simulink model "Swarm_Robot_Base_2017b"  (R2017b)
settings: Solver=VariableStepAuto  StartTime=0.0  StopTime=20  FixedStep=0.1  RelTol=1e-3
settings Model: Creator=jfu1  LastModifiedBy=Max
settings CodeAppCC: StateflowObjectComments=on

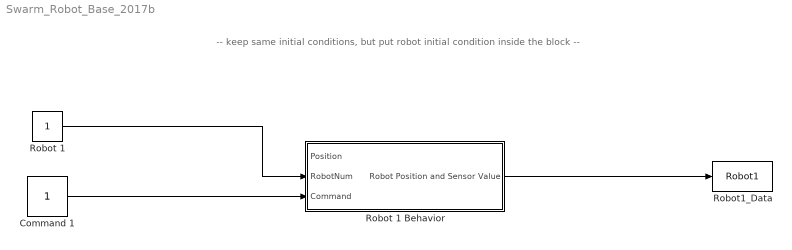
== system Swarm_Robot_Base_2017b ==
  note: -- keep same initial conditions, but put robot initial condition inside the block --
  Command 1 : Constant  VectorParams1D=off  SampleTime=-1
  Robot 1 : Constant
  Robot 1 Behavior : Subsystem
  Robot1_Data : ToWorkspace  VariableName=Robot1  SaveFormat=Timeseries  SampleTime=-1
  wires:
  Robot 1/1 -> Robot 1 Behavior/2(RobotNum)
  Command 1/1 -> Robot 1 Behavior/3(Command)
  Robot 1 Behavior/1("Robot Position and Sensor Value ") -> Robot1_Data/1

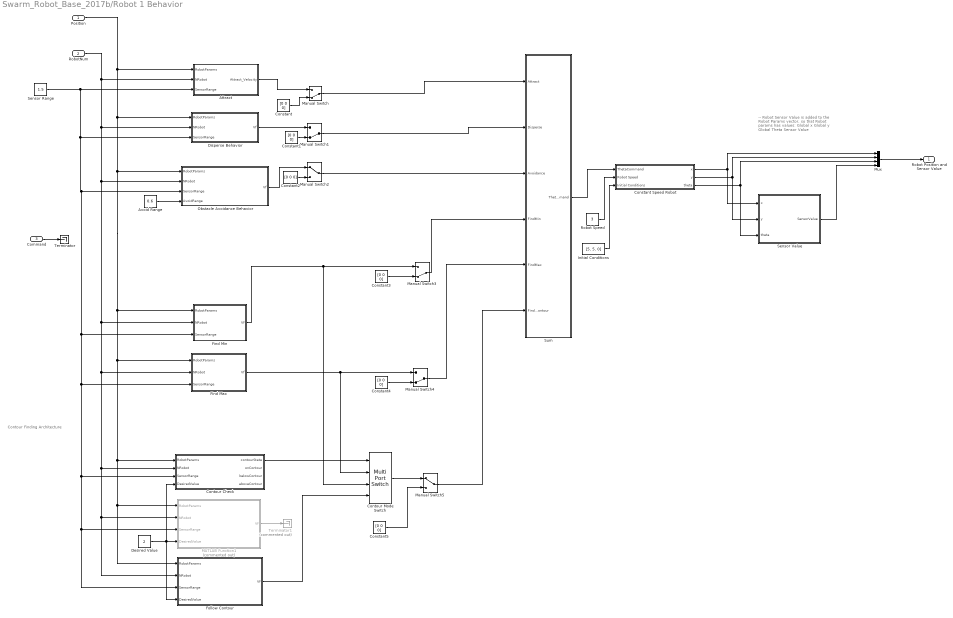
== system Swarm_Robot_Base_2017b/Robot 1 Behavior ==
  note: Contour Finding Architecture
  note: -- Robot Sensor Value is added
      | to the Robot Params vector, so that
      | Robot params has values:
      |           Global x
      |           Global y
      |           Global Theta
      |           Sensor Value
  Position : Inport
  RobotNum : Inport  Port=2
  Command : Inport  Port=3
  Attract : MATLAB Function  TreatAsAtomicUnit=on
  Avoid Range : Constant  Value=0.6
  Constant{,1..5} (6 alike) : Constant  Value=[0 0 0]
  Constant Speed Robot : Subsystem
  Contour Check : MATLAB Function  TreatAsAtomicUnit=on
  Contour Mode Switch : MultiPortSwitch
  Desired Value : Constant  Value=2
  Disperse Behavior : MATLAB Function  TreatAsAtomicUnit=on
  Find Max : MATLAB Function  TreatAsAtomicUnit=on
  Find Min : MATLAB Function  TreatAsAtomicUnit=on
  Follow Contour : MATLAB Function  TreatAsAtomicUnit=on
  Initial Conditions : Constant  Value=[5, 5, 0]
  MATLAB Function1 : MATLAB Function  Commented=on  TreatAsAtomicUnit=on
  Manual Switch{,1,3..4} (4 alike) : ManualSwitch  CurrentSetting=0
  Manual Switch2 : ManualSwitch
  Manual Switch5 : ManualSwitch
  Mux : Mux
  Obstacle Avoidance Behavior : MATLAB Function  TreatAsAtomicUnit=on
  Robot Speed : Constant  Value=3
  Sensor Range : Constant  Value=1.5
  Sensor Value : MATLAB Function  TreatAsAtomicUnit=on
  Sum : MATLAB Function  TreatAsAtomicUnit=on
  Terminator : Terminator
  Terminator1 : Terminator  Commented=on
  "Robot Position and Sensor Value " : Outport
  wires:
  Obstacle Avoidance Behavior/1(Vf) -> Manual Switch2/1
  Position/1 -> Follow Contour/1(RobotParams), MATLAB Function1/1(RobotParams), Contour Check/1(RobotParams), Find Max/1(RobotParams), Find Min/1(RobotParams), Obstacle Avoidance Behavior/1(RobotParams), Disperse Behavior/1(RobotParams), Attract/1(RobotParams)
  Disperse Behavior/1(Vf) -> Manual Switch1/1
  Initial Conditions/1 -> Constant Speed Robot/3(Initial Conditions)
  Sensor Value/1(SensorValue) -> Mux/4
  Mux/1 -> "Robot Position and Sensor Value "/1
  Constant Speed Robot/1(x) -> Sensor Value/1(x), Mux/1
  Constant Speed Robot/2(y) -> Mux/2, Sensor Value/2(y)
  Constant Speed Robot/3(theta) -> Mux/3, Sensor Value/3(theta)
  Attract/1(Attract_Velocity) -> Manual Switch/1
  Sensor Range/1 -> Follow Contour/3(SensorRange), MATLAB Function1/3(SensorRange), Contour Check/3(SensorRange), Find Max/3(SensorRange), Find Min/3(SensorRange), Obstacle Avoidance Behavior/3(SensorRange), Disperse Behavior/3(SensorRange), Attract/3(SensorRange)
  Robot Speed/1 -> Constant Speed Robot/2(Robot Speed)
  Sum/1(ThetaCommand) -> Constant Speed Robot/1(ThetaCommand)
  Manual Switch/1 -> Sum/1(Attract)
  Constant/1 -> Manual Switch/2
  Constant1/1 -> Manual Switch1/2
  Manual Switch1/1 -> Sum/2(Disperse)
  Avoid Range/1 -> Obstacle Avoidance Behavior/4(AvoidRange)
  Constant2/1 -> Manual Switch2/2
  Manual Switch2/1 -> Sum/3(Avoidance)
  Constant3/1 -> Manual Switch3/2
  Find Min/1(Vf) -> Contour Mode Switch/3, Manual Switch3/1
  Manual Switch3/1 -> Sum/4(FindMin)
  Constant4/1 -> Manual Switch4/2
  Find Max/1(Vf) -> Contour Mode Switch/2, Manual Switch4/1
  Command/1 -> Terminator/1
  RobotNum/1 -> Obstacle Avoidance Behavior/2(NRobot), Follow Contour/2(NRobot), MATLAB Function1/2(NRobot), Contour Check/2(NRobot), Find Max/2(NRobot), Find Min/2(NRobot), Disperse Behavior/2(NRobot), Attract/2(NRobot)
  Desired Value/1 -> Follow Contour/4(DesiredValue), Contour Check/4(DesiredValue), MATLAB Function1/4(DesiredValue)
  Manual Switch5/1 -> Sum/6(FindContour)
  Constant5/1 -> Manual Switch5/2
  Manual Switch4/1 -> Sum/5(FindMax)
  Follow Contour/1(Vf) -> Contour Mode Switch/4
  Contour Mode Switch/1 -> Manual Switch5/1
  MATLAB Function1/1(Vf) -> Terminator1/1
  Contour Check/1(contourState) -> Contour Mode Switch/1

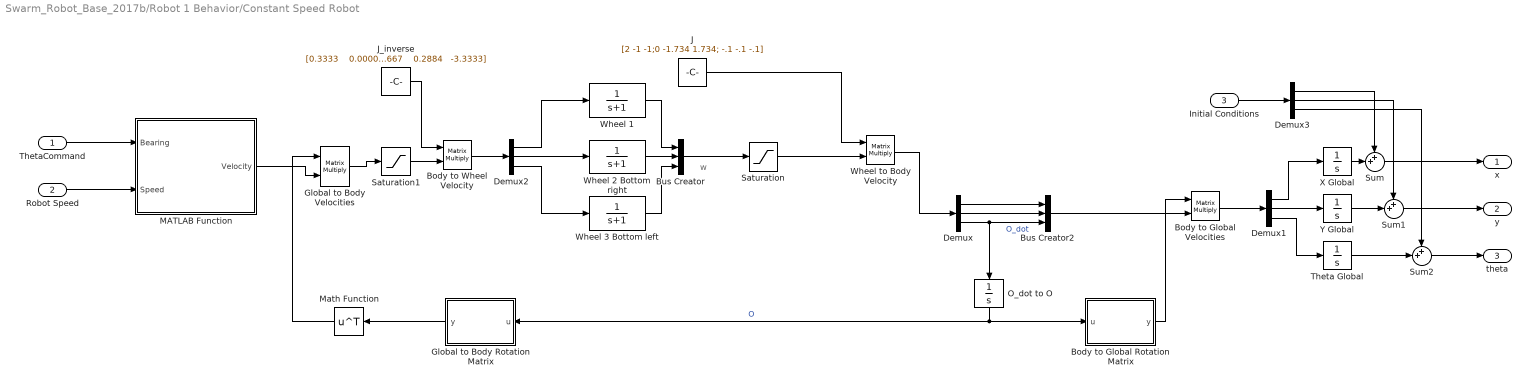
== system Swarm_Robot_Base_2017b/Robot 1 Behavior/Constant Speed Robot ==
  note: w
  ThetaCommand : Inport
  Robot Speed : Inport  Port=2
  Initial Conditions : Inport  Port=3
  Body to Global Velocities : Product  Multiplication=Matrix(*)
  Body to Global Rotation Matrix : MATLAB Function  TreatAsAtomicUnit=on
  Body to Wheel Velocity : Product  Multiplication=Matrix(*)
  Bus Creator : BusCreator  Inputs=3
  Bus Creator2 : BusCreator  Inputs=3
  Demux{,1..3} (4 alike) : Demux  Outputs=3
  Global to Body Velocities : Product  Multiplication=Matrix(*)
  Global to Body Rotation Matrix : MATLAB Function  TreatAsAtomicUnit=on
  J : Constant  Value=[2 -1 -1;0 -1.734 1.734; -.1 -.1 -.1]
  J_inverse : Constant  Value=|
      | [0.3333    0.0000   -3.3333
      |  ;  -0.1667   -0.2884   -3.3333
      |  ;  -0.1667    0.2884   -3.3333]
  MATLAB Function : MATLAB Function  TreatAsAtomicUnit=on
  Math Function : Math  Operator=transpose  SaturateOnIntegerOverflow=on
  O_dot to O : Integrator
  Saturation : Saturate  UpperLimit=6.28  LowerLimit=-6.28
  Saturation1 : Saturate  UpperLimit=2  LowerLimit=-2
  Sum : Sum  Inputs=++|
  Sum1 : Sum  Inputs=++|
  Sum2 : Sum  Inputs=++|
  Theta Global : Integrator
  Wheel 1 : TransferFcn  Denominator=[1 1]
  Wheel 2 Bottom right : TransferFcn  Denominator=[1 1]
  Wheel 3 Bottom left : TransferFcn  Denominator=[1 1]  ContinuousStateAttributes='orientation'
  Wheel to Body Velocity : Product  Multiplication=Matrix(*)
  X Global : Integrator
  Y Global : Integrator
  x : Outport
  y : Outport  Port=2
  theta : Outport  Port=3
  wires:
  Saturation/1 -> Wheel to Body Velocity/2
  Demux/1 -> Bus Creator2/1
  Demux2/1 -> Wheel 1/1
  Bus Creator/1 -> Saturation/1
  J_inverse/1 -> Body to Wheel Velocity/1
  Wheel to Body Velocity/1 -> Demux/1
  Bus Creator2/1 -> Body to Global Velocities/2
  Global to Body Velocities/1 -> Saturation1/1
  O_dot to O/1 -> Global to Body Rotation Matrix/1(u), Body to Global Rotation Matrix/1(u)  "O"
  Saturation1/1 -> Body to Wheel Velocity/2
  Body to Wheel Velocity/1 -> Demux2/1
  Wheel 1/1 -> Bus Creator/1
  Demux2/2 -> Wheel 2 Bottom right/1
  J/1 -> Wheel to Body Velocity/1
  Body to Global Rotation Matrix/1(y) -> Body to Global Velocities/1
  Demux/3 -> O_dot to O/1, Bus Creator2/3  "O_dot"
  Wheel 3 Bottom left/1 -> Bus Creator/3
  Demux2/3 -> Wheel 3 Bottom left/1
  Demux/2 -> Bus Creator2/2
  Wheel 2 Bottom right/1 -> Bus Creator/2
  Body to Global Velocities/1 -> Demux1/1
  Demux1/1 -> X Global/1
  Demux1/2 -> Y Global/1
  X Global/1 -> Sum/2
  Y Global/1 -> Sum1/2
  Demux1/3 -> Theta Global/1
  Initial Conditions/1 -> Demux3/1
  Demux3/1 -> Sum/1
  Sum/1 -> x/1
  Demux3/2 -> Sum1/1
  Theta Global/1 -> Sum2/2
  Demux3/3 -> Sum2/1
  Sum2/1 -> theta/1
  Sum1/1 -> y/1
  MATLAB Function/1(Velocity) -> Global to Body Velocities/2
  ThetaCommand/1 -> MATLAB Function/1(Bearing)
  Robot Speed/1 -> MATLAB Function/2(Speed)
  Global to Body Rotation Matrix/1(y) -> Math Function/1
  Math Function/1 -> Global to Body Velocities/1

== matlab function Swarm_Robot_Base_2017b/Robot 1 Behavior/Find Max ==
  data: RobotParams input; Vf output; NRobot input; SensorRange input
function Vf = FindMax(RobotParams, NRobot, SensorRange)
% calls the SwarmSimFindMax behavior

Vf= SwarmSimFindMax(RobotParams, NRobot, SensorRange);
end

== matlab function Swarm_Robot_Base_2017b/Robot 1 Behavior/MATLAB Function1 ==
  data: RobotParams input; Vf output; NRobot input; SensorRange input; DesiredValue input
function Vf   = Contour_Finding(RobotParams, NRobot, SensorRange, DesiredValue)

[Vf]  = SwarmSimFindContour(RobotParams, NRobot, SensorRange, DesiredValue);

end

== matlab function Swarm_Robot_Base_2017b/Robot 1 Behavior/Follow Contour ==
  data: RobotParams input; Vf output; NRobot input; SensorRange input; DesiredValue input
function Vf  = FollowContour(RobotParams, NRobot, SensorRange,  DesiredValue)
% calls the SwarmSimFollow behavior

[Vf] = SwarmSimFollowContour(RobotParams, NRobot, SensorRange, DesiredValue);

end

== matlab function Swarm_Robot_Base_2017b/Robot 1 Behavior/Contour Check ==
  data: contourState output; RobotParams input; NRobot input; SensorRange input; DesiredValue input; onContour output; belowContour output; aboveContour output
function [contourState, onContour, belowContour, aboveContour] = ContourCheck(RobotParams, NRobot, SensorRange,  DesiredValue)
% calls the SwarmSimOnContour behavior function

[contourState, onContour, belowContour, aboveContour] = SwarmSimOnContour(RobotParams, NRobot, SensorRange, DesiredValue);

end

== matlab function Swarm_Robot_Base_2017b/Robot 1 Behavior/Disperse Behavior ==
  data: Vf output; RobotParams input; NRobot input; SensorRange input
function Vf = disperse(RobotParams,NRobot,SensorRange)
Vf= SwarmSimDisperse(RobotParams, NRobot, SensorRange);
end

== matlab function Swarm_Robot_Base_2017b/Robot 1 Behavior/Obstacle Avoidance Behavior ==
  data: Vf output; RobotParams input; NRobot input; SensorRange input; AvoidRange input
function Vf = ObstacleAvoidance(RobotParams,NRobot, SensorRange, AvoidRange)

% This Matlab Function block calls the SwarmSimObstacleAvoid function. For
% details on function, see SwarmSimObstacleAvoid.m

[Vf] = SwarmSimObstacleAvoid(RobotParams, NRobot, SensorRange, AvoidRange); 
end

== matlab function Swarm_Robot_Base_2017b/Robot 1 Behavior/Sensor Value ==
  data: x input; SensorValue output; y input; theta input
function SensorValue = SensorValue_from_position(x, y, theta)
% this function determines the Sensor Value for the given robot for the
% desired concentration profile
 %%%%%%%%%%%%%%%%%%%%%%%%%%%%%%%%
 
 %NEED TO UPDATE TO CALL A FUNCTION 
 
 % from the 1x3 vector CurrentPosition, extract current global (x,y) and
 
 %note that in most applications theta will be unused

% given the current x,y position, determine the Sensor Value based off
% current (x,y) position

%To change the concentration profile, change here:

%concentration= sqrt(x^2 + y^2); %simple source function centered at origin

z= readScalarField(x,y);
SensorValue= z;

end

== matlab function Swarm_Robot_Base_2017b/Robot 1 Behavior/Find Min ==
  data: RobotParams input; Vf output; NRobot input; SensorRange input
function Vf = FindMin(RobotParams, NRobot, SensorRange)
% Matlab Function block calls the SwarmSimFindMin function 

Vf= SwarmSimFindMin(RobotParams, NRobot,SensorRange); 
end

== matlab function Swarm_Robot_Base_2017b/Robot 1 Behavior/Attract ==
  data: RobotParams input; Attract_Velocity output; NRobot input; SensorRange input
function Attract_Velocity = Attract(RobotParams, NRobot, SensorRange)
%calls the SwarmSimAttract function to determine robot velocities for
%attract behavior. 

Attract_Velocity = SwarmSimAttract(RobotParams,NRobot,SensorRange);

== matlab function Swarm_Robot_Base_2017b/Robot 1 Behavior/Sum ==
  data: Attract input; ThetaCommand output; Disperse input; Avoidance input; FindMin input; FindMax input; FindContour input
function ThetaCommand = VelocitySum(Attract,Disperse,Avoidance,FindMin,FindMax,FindContour)

% This Matlab Function block calls the SwarmSimSum function. For details on
% SwarmSimSum function, see SwarmSimSum.m

ThetaCommand = SwarmSimSum(Attract, Disperse, Avoidance, FindMin, FindMax, FindContour);
end

== matlab function Swarm_Robot_Base_2017b/Robot 1 Behavior/Constant Speed Robot/Body to Global Rotation Matrix ==
  data: u input; y output
function y = fcn(u)

y = [cos(u) -sin(u) 0; sin(u) cos(u) 0; 0 0 1];

== matlab function Swarm_Robot_Base_2017b/Robot 1 Behavior/Constant Speed Robot/Global to Body Rotation Matrix ==
  data: u input; y output
function y = fcn(u)

y = [cos(u) -sin(u) 0; sin(u) cos(u) 0; 0 0 1];

%y= [cos(u) sin(u) 0; -sin(u) cos(u) 0; 0 0 1]; 

% y= A';

== matlab function Swarm_Robot_Base_2017b/Robot 1 Behavior/Constant Speed Robot/MATLAB Function ==
  data: Bearing input; Speed input; Velocity output
function Velocity = rob_vel_from_bearing(Bearing, Speed)
% function block calculates robot velocity based off user-set constant
% robot velocity and bearing calculated from behaviors.

if Bearing == NaN;
    Vx= 0 ;
    Vy= 0;
    Vt= 0;
else
    Vx= Speed*cos(Bearing);
    Vy= Speed*sin(Bearing);
    Vt= 0.0;
end

Velocity = [Vx ; Vy ; Vt];
end
